simulink model "OCT_array_ready"  (R2018b)
settings: Solver=ode15s  StartTime=0.0  StopTime=sim_time  MaxStep=5  RelTol=1e-3  AbsTol=1e-3
values from neighbouring files (symbols this model uses):
  flow = sqrt(k_scale)*nom_flow    [ayazParams_init.m]    (also in multinode_wing_tail.m)
  set_alti = k_scale*set_alti_nom    (= 20)    [ayazParams_init.m]    (also in multinode_wing_tail.m = 200)
  set_pitch = set_pitch*(pi/180)    (= 0.12217304764)    [ayazParams_init.m]    (also in multinode_wing_tail.m)
  unstretched_l = unstretched_l - ini_elongation - added_elongation    [ayazParams_init.m]    (also in multinode_wing_tail.m)
  X0 = cat(1,ini_Rcm_o,ini_O_Vcm_o,ini_euler_ang,ini_OwB,ini_platform_ang,ini_platform_vel,     ini_R1i_o,ini_R2i_o,ini_R3i_o,ini_O_V1i_o,ini_O_V2i_o,ini_O_V3i_o)    [ayazParams_init.m]    (also in multinode_wing_tail.m)
settings Model: Creator=Ayaz  LastModifiedBy=Ayaz

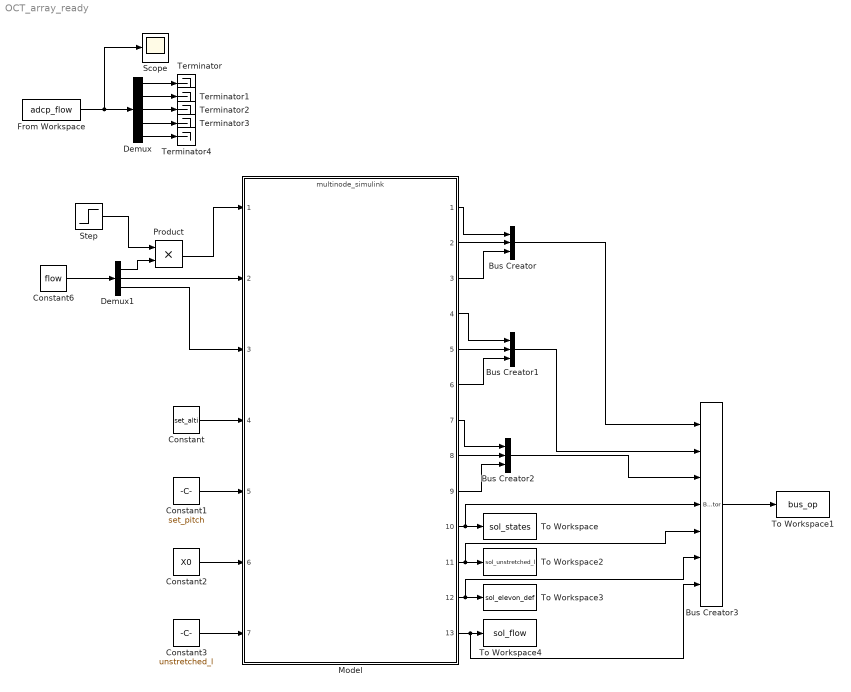
== system OCT_array_ready ==
  Bus Creator : BusCreator  Inputs=3
  Bus Creator1 : BusCreator  Inputs=3
  Bus Creator2 : BusCreator  Inputs=3
  Bus Creator3 : BusCreator  Inputs=7
  Constant : Constant  Value=set_alti
  Constant1 : Constant  Value=set_pitch
  Constant2 : Constant  Value=X0
  Constant3 : Constant  Value=unstretched_l
  Constant6 : Constant  Value=flow
  Demux : Demux  Outputs=5
  Demux1 : Demux  Outputs=3
  From Workspace : FromWorkspace  VariableName=adcp_flow  SampleTime=0
  Model : ModelReference  ModelNameDialog=multinode_simulink  SimulationMode=Normal  ModelReferenceVersion=1.312
  Product : Product
  Scope : Scope
  Step : Step  Time=0  SampleTime=0
  Terminator{,1..4} (5 alike) : Terminator
  To Workspace : ToWorkspace  VariableName=sol_states  SaveFormat=Timeseries  SampleTime=-1
  To Workspace1 : ToWorkspace  VariableName=bus_op  SaveFormat=Timeseries  SampleTime=-1
  To Workspace2 : ToWorkspace  VariableName=sol_unstretched_l  SaveFormat=Timeseries  SampleTime=-1
  To Workspace3 : ToWorkspace  VariableName=sol_elevon_def  SaveFormat=Timeseries  SampleTime=-1
  To Workspace4 : ToWorkspace  VariableName=sol_flow  SaveFormat=Timeseries  SampleTime=-1
  wires:
  Model/1 -> Bus Creator/1
  Model/2 -> Bus Creator/2
  Model/3 -> Bus Creator/3
  Model/4 -> Bus Creator1/1
  Model/5 -> Bus Creator1/2
  Model/6 -> Bus Creator1/3
  Model/10 -> To Workspace/1, Bus Creator3/4
  Model/11 -> Bus Creator3/5, To Workspace2/1
  Model/12 -> To Workspace3/1, Bus Creator3/6
  Model/9 -> Bus Creator2/3
  Model/8 -> Bus Creator2/2
  Model/7 -> Bus Creator2/1
  Model/13 -> Bus Creator3/7, To Workspace4/1
  Bus Creator/1 -> Bus Creator3/1
  Bus Creator1/1 -> Bus Creator3/2
  Bus Creator2/1 -> Bus Creator3/3
  Bus Creator3/1 -> To Workspace1/1
  From Workspace/1 -> Scope/1, Demux/1
  Constant3/1 -> Model/7
  Constant2/1 -> Model/6
  Constant1/1 -> Model/5
  Constant/1 -> Model/4
  Demux1/2 -> Model/2
  Demux1/3 -> Model/3
  Demux/1 -> Terminator/1
  Demux/2 -> Terminator1/1
  Demux/3 -> Terminator2/1
  Demux/4 -> Terminator3/1
  Demux/5 -> Terminator4/1
  Constant6/1 -> Demux1/1
  Demux1/1 -> Product/2
  Product/1 -> Model/1
  Step/1 -> Product/1
